simulink model "linear_ADRC"  (R2018b)
settings: Solver=VariableStepAuto  StartTime=0.0  StopTime=300  RelTol=1e-3
InitFcn:
  | %%%%%%%%%%%%%%%%%%%%%%%%%
  | %                     TUNABLE PARAMETERS                 %
  | %    (ORDER, SETTLING TIME, ESO GAIN AND B0)  %
  | %%%%%%%%%%%%%%%%%%%%%%%%%
  | order = 4;                     % ADRC order
  | ts = 3;                        % Desired settling time
  | b0 = 3;                         % b0 parameter
  | eso_gain = 15;                % ESO Dynamic related to closed-loop poles
  | 
  | %%%%%%%%%%%%%%%%%%%%%%%%%
  | %                                 ADRC                               %
  | %      (CONTROLLER GAINS AND ESO MATRIXES)    %
  | %%%%%%%%%%%%%%%%%%%%%%%%%
  | s_cl = 4/ts;                           % Closed-loop system poles
  | s_eso = eso_gain * s_cl;        % ESO poles
  | pole = [1 s_cl];                     % Base polynomial to calculate
  |                                            % System characteristic polynomial
  | pole_eso = [1 s_eso];            % Base polynomial to calculate
  |                                            % ESO characteristic polynomial
  | A = zeros(order + 1);            % Matrix A of ESO
  | B = zeros(order + 1, 1);        % Matrix B of ESO
  | C = [1 zeros(1, order)];         % Matrix C of ESO
  | 
  | %%%%%%%%%%%%%%%%%%%%%%%%%%%%%%%%%%%
  | % Here we'll calculate the characteristic polynomials of system and ESO,   %
  | % starting with the base polynomial, and convoluting it until we achieve    %
  | % the system's order.                                                                           %
  | % Also, we'll put the values of A and B matrixes of ESO, filling the             %
  | % diagonal above the main diagonal of A with one's, and putting the value %
  | % b0 on the penultimate value of B matrix, according to ADRC generalized %
  | % model fot Nth order.                                                                          %
  | %%%%%%%%%%%%%%%%%%%%%%%%%%%%%%%%%%%
  | A_sys = pole;
  | A_eso = pole_eso;
  | 
  | for i = 1:order
  |     if i ~= order
  |         A_sys = conv(A_sys, pole);
  |     else
  |         B(i) = b0;
  |     end
  |     A(i,i+1) = 1;
  |     A_eso = conv(A_eso, pole_eso);
  | end
  | 
  | K = [1 A_sys(2:end)];           % Controller gain matrix
  | L = A_eso(2:end)';               % ESO gain matrix
undefined symbols (not defined in the file or in its folder): As, B1, B2, Cs
libraries: dspindex x1
settings Model: Creator=leony  LastModifiedBy=root
settings DebuggingCC: LibraryContextMissingDiagnostic=none
settings SFSimCC: SimUseLocalCustomCode=off
settings RTWCC: RTWUseLocalCustomCode=off

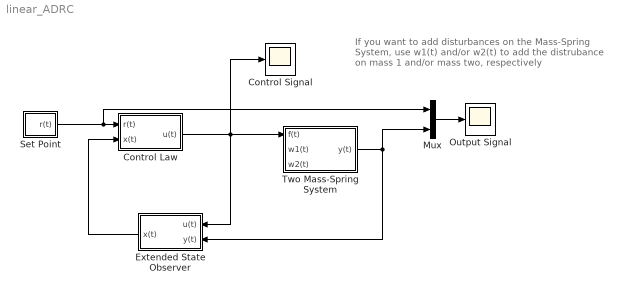
== system linear_ADRC ==
  note: If you want to add disturbances on the Mass-Spring System, use w1(t) and/or w2(t) to add the distrubance on mass 1 and/or mass two, respectively
  Control Law : Subsystem
  Control Signal : Scope
  Extended State Observer : Subsystem
  Mux : Mux  Inputs=2
  Output Signal : Scope
  Set Point : Subsystem
  "Two Mass-Spring System " : Subsystem
  wires:
  Mux/1 -> Output Signal/1
  Control Law/1(u(t)) -> Control Signal/1, "Two Mass-Spring System "/1(f(t)), Extended State Observer/1("u(t) ")
  Extended State Observer/1(x(t)) -> Control Law/2(x(t))
  "Two Mass-Spring System "/1(y(t)) -> Mux/2, Extended State Observer/2(y(t))
  Set Point/1(r(t)) -> Mux/1, Control Law/1(r(t))

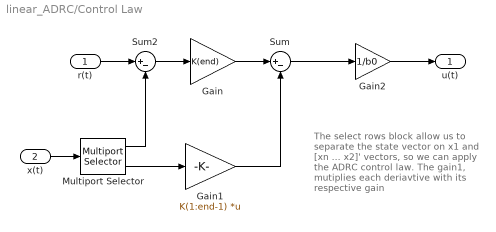
== system linear_ADRC/Control Law ==
  note: The select rows block allow us to separate the state vector on x1 and [xn ... x2]' vectors, so we can apply the ADRC control law. The gain1, mutiplies each deriavtive with its respective gain
  r(t) : Inport
  x(t) : Inport  Port=2
  Gain : Gain  Gain=K(end)  ParamDataTypeStr=Inherit: Inherit from 'Gain'
  Gain1 : Gain  Gain=K(1:end-1)  Multiplication=Matrix(K*u) (u vector)
  Gain2 : Gain  Gain=1/b0
  Multiport Selector : dspindex/Multiport Selector  rowsOrCols=Rows  idxCellArray={ 1, [order+1:-1:2]}  idxErrMode=Clip Index
  Sum : Sum  Inputs=|+-
  Sum2 : Sum  Inputs=|+-
  u(t) : Outport
  wires:
  Gain2/1 -> u(t)/1
  Sum/1 -> Gain2/1
  r(t)/1 -> Sum2/1
  Sum2/1 -> Gain/1
  Gain/1 -> Sum/1
  x(t)/1 -> Multiport Selector/1
  Multiport Selector/1 -> Sum2/2
  Multiport Selector/2 -> Gain1/1
  Gain1/1 -> Sum/2

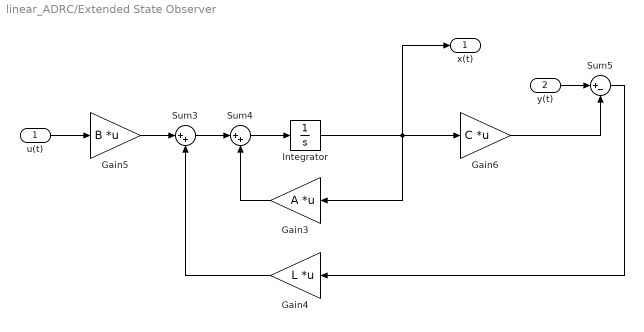
== system linear_ADRC/Extended State Observer ==
  "u(t) " : Inport
  y(t) : Inport  Port=2
  Gain3 : Gain  Gain=A  Multiplication=Matrix(K*u) (u vector)
  Gain4 : Gain  Gain=L  Multiplication=Matrix(K*u) (u vector)
  Gain5 : Gain  Gain=B  Multiplication=Matrix(K*u) (u vector)
  Gain6 : Gain  Gain=C  Multiplication=Matrix(K*u) (u vector)
  Integrator : Integrator
  Sum3 : Sum  Inputs=|++
  Sum4 : Sum  Inputs=|++
  Sum5 : Sum  Inputs=|+-
  x(t) : Outport
  wires:
  Sum4/1 -> Integrator/1
  y(t)/1 -> Sum5/1
  Gain4/1 -> Sum3/2
  Gain5/1 -> Sum3/1
  Gain3/1 -> Sum4/2
  Sum3/1 -> Sum4/1
  Sum5/1 -> Gain4/1
  Gain6/1 -> Sum5/2
  Integrator/1 -> x(t)/1, Gain3/1, Gain6/1
  "u(t) "/1 -> Gain5/1

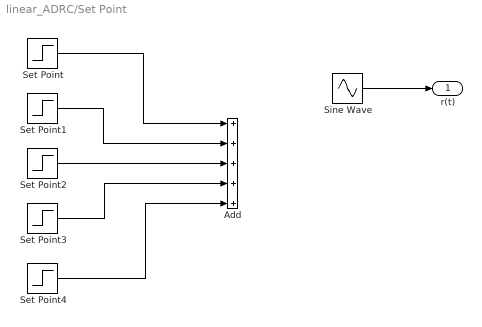
== system linear_ADRC/Set Point ==
  Add : Sum  Inputs=+++++
  Set Point : Step  Time=0  SampleTime=0
  Set Point1 : Step  Time=50  After=0.8  SampleTime=0
  Set Point2 : Step  Time=120  After=-1.3  SampleTime=0
  Set Point3 : Step  Time=180  After=0.5  SampleTime=0
  Set Point4 : Step  Time=250  After=0.4  SampleTime=0
  Sine Wave : Sin  Amplitude=3  SampleTime=0
  r(t) : Outport
  wires:
  Set Point2/1 -> Add/3
  Set Point4/1 -> Add/5
  Set Point3/1 -> Add/4
  Set Point1/1 -> Add/2
  Set Point/1 -> Add/1
  Sine Wave/1 -> r(t)/1

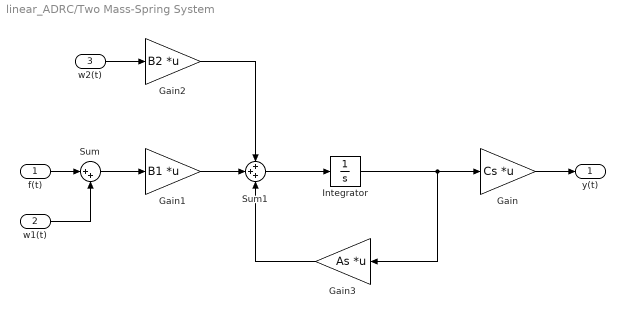
== system linear_ADRC/Two Mass-Spring System  ==
  f(t) : Inport
  w1(t) : Inport  Port=2
  w2(t) : Inport  Port=3
  Gain : Gain  Gain=Cs  Multiplication=Matrix(K*u) (u vector)
  Gain1 : Gain  Gain=B1  Multiplication=Matrix(K*u) (u vector)
  Gain2 : Gain  Gain=B2  Multiplication=Matrix(K*u) (u vector)
  Gain3 : Gain  Gain=As  Multiplication=Matrix(K*u) (u vector)
  Integrator : Integrator
  Sum : Sum  Inputs=|++
  Sum1 : Sum  Inputs=+++
  y(t) : Outport
  wires:
  Gain/1 -> y(t)/1
  Integrator/1 -> Gain3/1, Gain/1
  f(t)/1 -> Sum/1
  Sum/1 -> Gain1/1
  Gain1/1 -> Sum1/2
  Gain3/1 -> Sum1/3
  Sum1/1 -> Integrator/1
  Gain2/1 -> Sum1/1
  w2(t)/1 -> Gain2/1
  w1(t)/1 -> Sum/2
